simulink model "Proporcional_simu"  (R2021a)
settings: Solver=VariableStepAuto  StartTime=0.0  StopTime=5  RelTol=1e-3
values from neighbouring files (symbols this model uses):
  x0 = [pos0 0 0 0]    [proporcional.m]
undefined symbols (not defined in the file or in its folder): Ass, Bss, Css, Dss
libraries: cstblocks x1
settings Model: Creator=Santiago  LastModifiedBy=Santiago

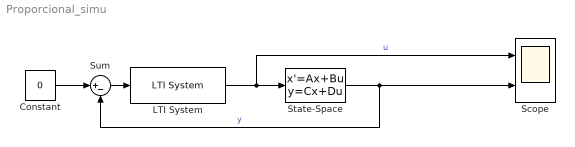
== system Proporcional_simu ==
  Constant : Constant  Value=0
  LTI System : cstblocks/LTI System  sys=Cd  IC=[]
  Scope : Scope  NumInputPorts=2
  State-Space : StateSpace  A=Ass  B=Bss  C=Css  D=Dss  InitialCondition=x0  ParameterTunability=Unconstrained
  Sum : Sum  Inputs=|+-
  wires:
  LTI System/1 -> State-Space/1, Scope/1  "u"
  Sum/1 -> LTI System/1
  Constant/1 -> Sum/1
  State-Space/1 -> Sum/2, Scope/2  "y"
